simulink model "RB_KAIROS_impControl_repulsive"  (R2020b)
settings: Solver=ode4  StartTime=0.0  StopTime=t_end  FixedStep=Ts  RelTol=1e-3
values from neighbouring files (symbols this model uses):
  am = 0.3    [RB_KAIROS_ImpControl_OpSpace_quat_2020b_safety_main.m]
  am_r = 0.3    [RB_KAIROS_ImpControl_OpSpace_quat_2020b_safety_main.m]
  Kc = diag(50*ones(6,1))    [RB_KAIROS_ImpControl_OpSpace_quat_2020b_safety_main.m]
  Kp = 2*[400;400;400;400;0;0;0]    [RB_KAIROS_ImpControl_OpSpace_quat_2020b_safety_main.m]
  Kv = [1000;1000;1000;[300;300;300;300;300;300;300]]    [RB_KAIROS_ImpControl_OpSpace_quat_2020b_safety_main.m]
  model_sample_time = 0.001    [RB_KAIROS_ImpControl_OpSpace_quat_2020b_safety_main.m]
  q_dot_0 = zeros(10,1)    [RB_KAIROS_ImpControl_OpSpace_quat_2020b_safety_main.m]
  T_i = K    [RB_KAIROS_ImpControl_OpSpace_quat_2020b_safety_main.m]
  tau_ext = [0 0 0 0 0 0 0 0 0 0 0]    [RB_KAIROS_ImpControl_OpSpace_quat_2020b_safety_main.m]
  v_SMU = 10    [RB_KAIROS_ImpControl_OpSpace_quat_2020b_safety_main.m]
  vm = 0.5    [RB_KAIROS_ImpControl_OpSpace_quat_2020b_safety_main.m]
  vm_r = 0.5    [RB_KAIROS_ImpControl_OpSpace_quat_2020b_safety_main.m]
undefined symbols (not defined in the file or in its folder): DiscIntNeverNeededParam, magnitude, q_0, T_f
libraries: simulink x4, utils x4, transformations_lib x3
(part 2 of 17)

== system RB_KAIROS_impControl_repulsive/CONTROLLER /Kinematics and Dynamics/Kinematics - error representation ==
  qv : Inport
  qa : Inport  Port=2
  R_D_W_aug : Inport  Port=3
  x_dot_des : Inport  Port=4
  x_ddot_des : Inport  Port=5
  x_err : Inport  Port=6
  x_dot_err : Inport  Port=7
  qv_dot : Inport  Port=8
  qa_dot : Inport  Port=9
  Compute J_x_dot : Subsystem
  MATLAB Function1 : MATLAB Function  TreatAsAtomicUnit=on
  MATLAB Function2 : MATLAB Function  TreatAsAtomicUnit=on
  MATLAB Function3 : MATLAB Function  TreatAsAtomicUnit=on
  Terminator : Terminator
  Whole-Body Jacobian : MATLAB Function  TreatAsAtomicUnit=on
  J_x : Outport
  J_x_dot : Outport  Port=2
  vt : Outport  Port=3
  vt_dot : Outport  Port=4
  J_b : Outport  Port=5
  wires:
  qa/1 -> Compute J_x_dot/5(qa), Whole-Body Jacobian/2(qa)
  qv/1 -> Compute J_x_dot/4(qv), Whole-Body Jacobian/1(qv)
  Whole-Body Jacobian/1(J) -> MATLAB Function3/2(J_b), MATLAB Function1/1(J), J_b/1, Compute J_x_dot/1(J_b)
  MATLAB Function3/1(J_x) -> J_x/1
  Compute J_x_dot/1(J_x_dot) -> J_x_dot/1
  R_D_W_aug/1 -> MATLAB Function3/1(R_W_D_aug), Compute J_x_dot/2(R_D_W_aug), MATLAB Function2/1(R_D_W_aug)
  x_dot_des/1 -> Compute J_x_dot/3(x_dot_d), MATLAB Function2/2(x_dot_d)
  MATLAB Function2/2(vt_dot) -> vt_dot/1
  MATLAB Function2/1(vt) -> vt/1
  x_ddot_des/1 -> MATLAB Function2/3(x_ddot_d)
  x_dot_err/1 -> MATLAB Function2/5(x_dot_err)
  x_err/1 -> MATLAB Function2/4(x_err)
  MATLAB Function1/1(t) -> Terminator/1
  qv_dot/1 -> Compute J_x_dot/6(qv_dot)
  qa_dot/1 -> Compute J_x_dot/7(qa_dot)

== system RB_KAIROS_impControl_repulsive/Trajectory Generator/Subsystem1/Angle Axis Via Quaternions ==
  R : Inport
  Display : Display
  Quaternion To Angle Axis : Subsystem
  Reshape : Reshape  OutputDimensionality=Column vector (2-D)
  Selector : Selector  InputPortWidth=4  IndexOptions=Index vector (dialog)  Indices=2:4  OutputSizes=1
  Selector1 : Selector  InputPortWidth=4  IndexOptions=Index vector (dialog)  Indices=1  OutputSizes=1
  r2q : MATLAB Function  TreatAsAtomicUnit=on
  angle : Outport  VectorParamsAs1DForOutWhenUnconnected=off
  axis : Outport  Port=2  VectorParamsAs1DForOutWhenUnconnected=off
  wires:
  Quaternion To Angle Axis/2(axis) -> axis/1
  R/1 -> r2q/1(R)
  Quaternion To Angle Axis/1(angle) -> angle/1
  Selector/1 -> Reshape/1
  Selector1/1 -> Quaternion To Angle Axis/1(eta)
  r2q/1(q) -> Selector1/1, Selector/1
  Reshape/1 -> Display/1, Quaternion To Angle Axis/2(epsilon)

== system RB_KAIROS_impControl_repulsive/Trajectory Generator/Subsystem1/Normalize ==
  x : Inport
  Divide : Product  Inputs=*/
  Switch : Switch  Criteria=u2 > Threshold
  length : Subsystem
  one : Constant
  x/||x|| : Outport  VectorParamsAs1DForOutWhenUnconnected=off
  wires:
  x/1 -> Divide/1, length/1(v)
  Divide/1 -> x/||x||/1
  one/1 -> Switch/3
  length/1(|v|) -> Switch/2, Switch/1
  Switch/1 -> Divide/2

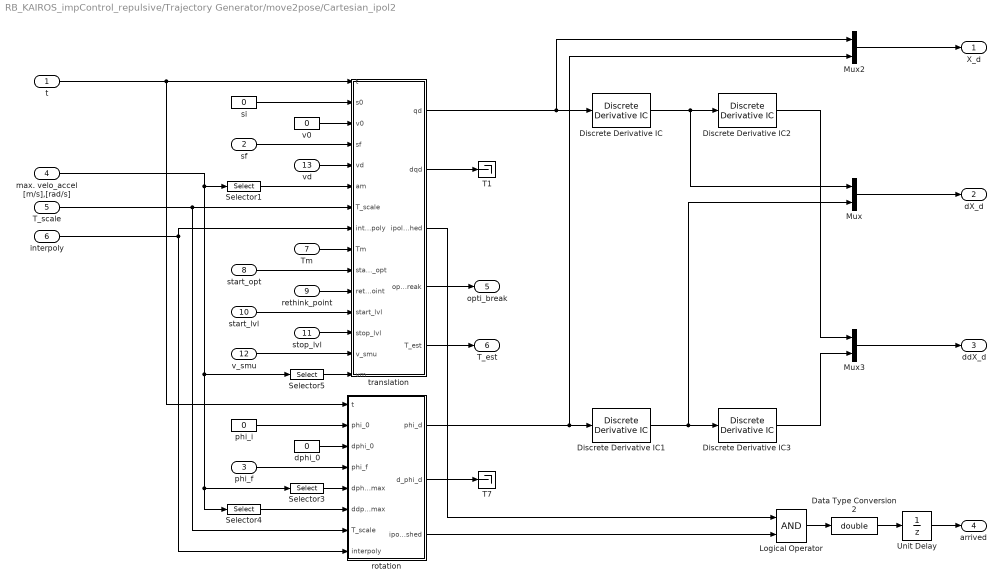
== system RB_KAIROS_impControl_repulsive/Trajectory Generator/move2pose/Cartesian_ipol2 ==
  t : Inport
  sf : Inport  Port=2
  phi_f : Inport  Port=3
  max. velo_accel [m/s],[rad/s] : Inport  Port=4
  T_scale : Inport  Port=5
  interpoly : Inport  Port=6
  Tm : Inport  Port=7
  start_opt : Inport  Port=8
  rethink_point : Inport  Port=9
  start_lvl : Inport  Port=10
  stop_lvl : Inport  Port=11
  v_smu : Inport  Port=12
  vd : Inport  Port=13
  Data Type Conversion2 : DataTypeConversion  OutDataTypeStr=double
  Discrete Derivative IC{,1..3} (4 alike) : utils/Discrete Derivative IC  model_sample_time=model_sample_time
  Logical Operator : Logic  AllPortsSameDT=off  OutDataTypeStr=boolean
  Mux : Mux  Inputs=2
  Mux2 : Mux  Inputs=2
  Mux3 : Mux  Inputs=2
  Selector1 : Selector  InputPortWidth=4  IndexOptions=Index vector (dialog)  Indices=2  OutputSizes=1
  Selector3 : Selector  InputPortWidth=4  IndexOptions=Index vector (dialog)  Indices=3  OutputSizes=1
  Selector4 : Selector  InputPortWidth=4  IndexOptions=Index vector (dialog)  Indices=4  OutputSizes=1
  Selector5 : Selector  InputPortWidth=4  IndexOptions=Index vector (dialog)  Indices=1  OutputSizes=1
  T1 : Terminator
  T7 : Terminator
  Unit Delay : UnitDelay  SampleTime=-1  HasFrameUpgradeWarning=on
  dphi_0 : Constant  Value=0
  phi_i : Constant  Value=0
  rotation : Subsystem
  si : Constant  Value=0
  translation : Subsystem
  v0 : Constant  Value=0
  X_d : Outport  VectorParamsAs1DForOutWhenUnconnected=off
  dX_d : Outport  Port=2  VectorParamsAs1DForOutWhenUnconnected=off
  ddX_d : Outport  Port=3  VectorParamsAs1DForOutWhenUnconnected=off
  arrived : Outport  Port=4  VectorParamsAs1DForOutWhenUnconnected=off
  opti_break : Outport  Port=5  VectorParamsAs1DForOutWhenUnconnected=off
  T_est : Outport  Port=6  VectorParamsAs1DForOutWhenUnconnected=off
  wires:
  sf/1 -> translation/4(sf)
  Selector1/1 -> translation/6(am)
  max. velo_accel [m/s],[rad/s]/1 -> Selector4/1, Selector3/1, Selector5/1, Selector1/1
  Data Type Conversion2/1 -> Unit Delay/1
  dphi_0/1 -> rotation/3(dphi_0)
  Selector3/1 -> rotation/5(dphi_max)
  Selector4/1 -> rotation/6(ddphi_max)
  v0/1 -> translation/3(v0)
  Mux/1 -> dX_d/1
  t/1 -> rotation/1(t), translation/1(t)
  rotation/1(phi_d) -> Discrete Derivative IC1/1, Mux2/2
  T_scale/1 -> rotation/7(T_scale), translation/7(T_scale)
  interpoly/1 -> rotation/8(interpoly), translation/8(interpoly)
  Discrete Derivative IC/1 -> Mux/1, Discrete Derivative IC2/1
  Unit Delay/1 -> arrived/1
  translation/3(ipol_finished) -> Logical Operator/1
  Logical Operator/1 -> Data Type Conversion2/1
  Mux2/1 -> X_d/1
  translation/1(qd) -> Discrete Derivative IC/1, Mux2/1
  Mux3/1 -> ddX_d/1
  Discrete Derivative IC2/1 -> Mux3/1
  Discrete Derivative IC3/1 -> Mux3/2
  Discrete Derivative IC1/1 -> Discrete Derivative IC3/1, Mux/2
  rotation/3(ipol_finished) -> Logical Operator/2
  Tm/1 -> translation/9(Tm)
  translation/4(opti_break) -> opti_break/1
  translation/5(T_est) -> T_est/1
  start_opt/1 -> translation/10(start_opt)
  rethink_point/1 -> translation/11(rethink_point)
  start_lvl/1 -> translation/12(start_lvl)
  stop_lvl/1 -> translation/13(stop_lvl)
  v_smu/1 -> translation/14(v_smu)
  phi_i/1 -> rotation/2(phi_0)
  phi_f/1 -> rotation/4(phi_f)
  rotation/2(d_phi_d) -> T7/1
  translation/2(dqd) -> T1/1
  Selector5/1 -> translation/15(vm)
  vd/1 -> translation/5(vd)
  si/1 -> translation/2(s0)

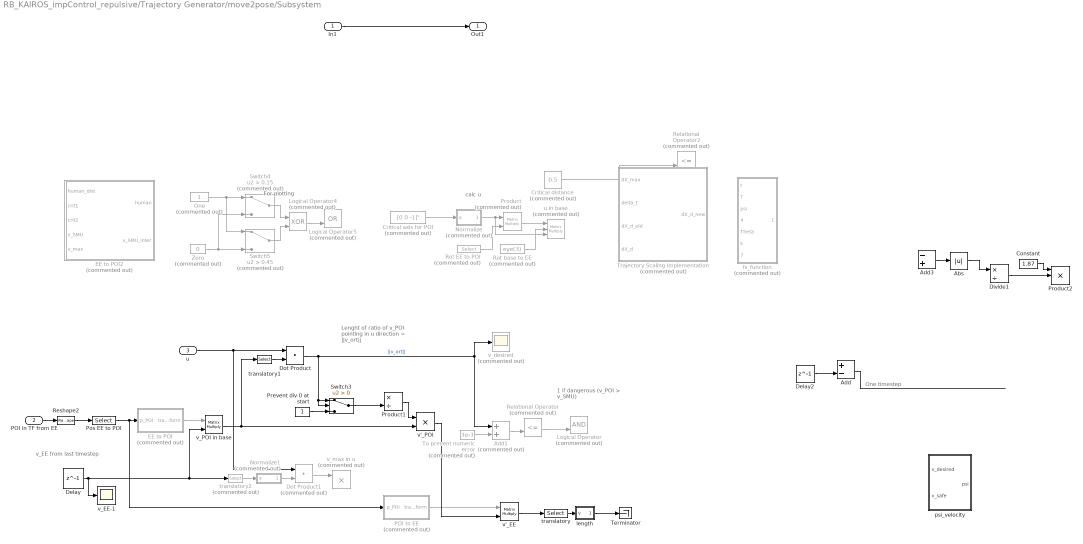
== system RB_KAIROS_impControl_repulsive/Trajectory Generator/move2pose/Subsystem ==
  note: calc u
  note: For plotting
  note: v_EE from last timestep
  note: 1 if dangerous
      | (v_POI > v_SMU)
  note: Lenght of ratio of v_POI
      | pointing in u direction
      | = ||v_ort||
  note: One timestep
  In1 : Inport
  POI in TF from EE : Inport  Port=2
  u : Inport  Port=3
  Abs : Abs
  Add : Sum  Inputs=+-
  Add1 : Sum  Commented=on
  Add3 : Sum  Inputs=-+
  Constant : Constant  Value=1.87
  Critical axis for POI : Constant  Commented=on  Value=[0 0 -1]'
  Critical distance : Constant  Commented=on  Value=0.5
  Delay : Delay  DelayLength=1
  Delay2 : Delay  DelayLength=1
  Divide1 : Product  Inputs=*/
  Dot Product : DotProduct  InputSameDT=on  OutDataTypeStr=Inherit: Inherit via internal rule
  Dot Product1 : DotProduct  Commented=on  InputSameDT=on  OutDataTypeStr=Inherit: Inherit via internal rule
  EE to POI : MATLAB Function  Commented=on  TreatAsAtomicUnit=on
  EE to POI2 : MATLAB Function  Commented=on  TreatAsAtomicUnit=on
  Logical Operator : Logic  Commented=on  AllPortsSameDT=off  OutDataTypeStr=boolean
  Logical Operator4 : Logic  Commented=on  Operator=XOR  AllPortsSameDT=off  OutDataTypeStr=boolean
  Logical Operator5 : Logic  Commented=on  Operator=OR  AllPortsSameDT=off  OutDataTypeStr=boolean
  Normalize : Subsystem  Commented=on
  Normalize1 : Subsystem  Commented=on
  One : Constant  Commented=on
  POI to EE : MATLAB Function  Commented=on  TreatAsAtomicUnit=on
  Pos EE to POI : Selector  NumberOfDimensions=2  InputPortWidth=7  IndexOptions=Index vector (dialog),Index vector (dialog)  Indices=[1:3],[4]  OutputSizes=1
  Prevent div 0 at start : Constant
  Product : Product  Commented=on  Multiplication=Matrix(*)
  Product1 : Product  Inputs=*/
  Product2 : Product  Inputs=3
  Relational Operator : RelationalOperator  Commented=on  Operator=<=  OutDataTypeStr=boolean  RndMeth=Simplest
  Relational Operator2 : RelationalOperator  Commented=on  Operator=<=  OutDataTypeStr=boolean  RndMeth=Simplest
  Reshape2 : Reshape  OutputDimensionality=Customize  OutputDimensions=[4,4]
  Rot EE to POI : Selector  Commented=on  NumberOfDimensions=2  InputPortWidth=7  IndexOptions=Index vector (dialog),Index vector (dialog)  Indices=[1:3],[1:3]  OutputSizes=1
  Rot base to EE : Constant  Commented=on  Value=eye(3)
  Switch3 : Switch  Criteria=u2 > Threshold
  Switch4 : Switch  Commented=on  Criteria=u2 > Threshold  Threshold=0.15
  Switch5 : Switch  Commented=on  Criteria=u2 > Threshold  Threshold=0.45
  Terminator : Terminator
  To prevent numeric error : Constant  Commented=on  Value=3e-3
  Trajectory Scaling Implementation : MATLAB Function  Commented=on  TreatAsAtomicUnit=on
  Zero : Constant  Commented=on  Value=0
  fs_function : MATLAB Function  Commented=on  TreatAsAtomicUnit=on
  length : Subsystem
  psi_velocity : MATLAB Function  TreatAsAtomicUnit=on
  translatory : Selector  InputPortWidth=6  IndexOptions=Index vector (dialog)  Indices=[1:3]  OutputSizes=1
  translatory1 : Selector  InputPortWidth=6  IndexOptions=Index vector (dialog)  Indices=[1:3]  OutputSizes=1
  translatory2 : Selector  Commented=on  InputPortWidth=6  IndexOptions=Index vector (dialog)  Indices=[1:3]  OutputSizes=1
  u in base : Product  Commented=on  Inputs=3  Multiplication=Matrix(*)
  v'_EE : Product  Multiplication=Matrix(*)
  v'_POI : Product
  v_EE-1 : Scope
  v_POI in base : Product  Multiplication=Matrix(*)
  v_desired : Scope  Commented=on
  v_max in u : Product  Commented=on
  Out1 : Outport  VectorParamsAs1DForOutWhenUnconnected=off
  wires:
  In1/1 -> Out1/1
  Critical axis for POI/1 -> Normalize/1(x)
  Rot EE to POI/1 -> Product/2
  Logical Operator4/1 -> Logical Operator5/2
  Product/1 -> u in base/1
  One/1 -> Switch4/1, Switch5/1
  Zero/1 -> Switch5/3, Switch4/3
  Switch4/1 -> Logical Operator4/1
  Switch5/1 -> Logical Operator4/2
  Normalize/1(x/||x||) -> u in base/3, Product/1
  Rot base to EE/1 -> u in base/2
  Critical distance/1 -> Relational Operator2/2
  Prevent div 0 at start/1 -> Switch3/3
  translatory2/1 -> Normalize1/1(x)
  Normalize1/1(x/||x||) -> Dot Product1/2
  ? -> Logical Operator/1
  ? -> v_max in u/2
  POI to EE/1(transform) -> v'_EE/1
  Add1/1 -> Relational Operator/2
  ? -> Product1/1
  v'_EE/1 -> translatory/1
  v'_POI/1 -> v'_EE/2
  EE to POI/1(transform) -> v_POI in base/1
  translatory/1 -> length/1(v)
  ? -> Relational Operator/1
  ? -> Delay/1
  v_POI in base/1 -> v'_POI/2, translatory1/1
  Dot Product1/1 -> v_max in u/1
  Delay/1 -> v_EE-1/1, v_POI in base/2, translatory2/1
  Dot Product/1 -> v_desired/1, Add1/1, Switch3/2, Switch3/1  "||v_ort||"
  translatory1/1 -> Dot Product/2
  Switch3/1 -> Product1/2
  Pos EE to POI/1 -> POI to EE/1(p_POI), EE to POI/1(p_POI)
  Reshape2/1 -> Pos EE to POI/1
  u/1 -> Dot Product/1, Dot Product1/1
  POI in TF from EE/1 -> Reshape2/1
  To prevent numeric error/1 -> Add1/2
  Product1/1 -> v'_POI/1
  length/1(|v|) -> Terminator/1
  Relational Operator/1 -> Logical Operator/2
  Delay2/1 -> Add/2
  ? -> Add/1
  ? -> Delay2/1
  Add/1 -> ?
  Abs/1 -> Divide1/1
  Constant/1 -> Product2/1
  Divide1/1 -> Product2/2
  Add3/1 -> Abs/1

== system RB_KAIROS_impControl_repulsive/CONTROLLER /Kinematics and Dynamics/Kinematics - error representation/Compute J_x_dot ==
  note: J_x_dot = R_D_W_aug*J_b_dot - R_D_W_aug*S(omega_d)_aug*J_b = R_D_W_aug*(J_b_dot - S(omega_d)_aug*J_b)
  J_b : Inport
  R_D_W_aug : Inport  Port=2
  x_dot_d : Inport  Port=3
  qv : Inport  Port=4
  qa : Inport  Port=5
  qv_dot : Inport  Port=6
  qa_dot : Inport  Port=7
  Add : Sum  Inputs=+-
  Augment matrix : MATLAB Function  TreatAsAtomicUnit=on
  MATLAB Function : MATLAB Function  TreatAsAtomicUnit=on
  MatrixMultiply : Product  Multiplication=Matrix(*)
  MatrixMultiply1 : Product  Multiplication=Matrix(*)
  S(omega) : MATLAB Function  TreatAsAtomicUnit=on
  Selector : Selector  InputPortWidth=6  IndexOptions=Index vector (dialog)  Indices=[4:6]  OutputSizes=1
  J_x_dot : Outport
  wires:
  Add/1 -> MatrixMultiply/2
  MATLAB Function/1(J_dot) -> Add/1
  MatrixMultiply1/1 -> Add/2
  x_dot_d/1 -> Selector/1
  Augment matrix/1(M_aug) -> MatrixMultiply1/1
  R_D_W_aug/1 -> MatrixMultiply/1
  qa_dot/1 -> MATLAB Function/4(qa_dot)
  Selector/1 -> S(omega)/1(v)
  S(omega)/1(S) -> Augment matrix/1(M)
  J_b/1 -> MatrixMultiply1/2
  qa/1 -> MATLAB Function/2(qa)
  qv_dot/1 -> MATLAB Function/3(qv_dot)
  MatrixMultiply/1 -> J_x_dot/1
  qv/1 -> MATLAB Function/1(qv)

== system RB_KAIROS_impControl_repulsive/Trajectory Generator/Subsystem1/Angle Axis Via Quaternions/Quaternion To Angle Axis ==
  eta : Inport
  epsilon : Inport  Port=2
  Divide : Product  Inputs=*/
  Gain : Gain  Gain=2
  Product : Product  RndMeth=Zero
  Saturation : Saturate  UpperLimit=1  LowerLimit=-1
  Sqrt : Sqrt  SaturateOnIntegerOverflow=on
  Subtract : Sum  Inputs=+-
  Switch1 : Switch  Criteria=u2 ~= 0
  Trigonometric Function : Trigonometry  Operator=acos
  dummy axis : Constant  Value=[1,0,0]
  one : Constant
  angle : Outport  VectorParamsAs1DForOutWhenUnconnected=off
  axis : Outport  Port=2  VectorParamsAs1DForOutWhenUnconnected=off
  wires:
  Divide/1 -> Switch1/1
  Switch1/1 -> axis/1
  dummy axis/1 -> Switch1/3
  Gain/1 -> Switch1/2, angle/1
  epsilon/1 -> Divide/1
  Trigonometric Function/1 -> Gain/1
  eta/1 -> Saturation/1
  Subtract/1 -> Sqrt/1
  one/1 -> Subtract/1
  Product/1 -> Subtract/2
  Sqrt/1 -> Divide/2
  Saturation/1 -> Trigonometric Function/1, Product/1, Product/2

== system RB_KAIROS_impControl_repulsive/Trajectory Generator/Subsystem1/Normalize/length ==
  v : Inport
  Abs1 : Abs
  Add : Sum  Inputs=+
  Math Function : Math  Operator=magnitude^2  SignedPower=on  SaturateOnIntegerOverflow=on
  Sqrt : Sqrt  Operator=signedSqrt  SaturateOnIntegerOverflow=on
  |v| : Outport  VectorParamsAs1DForOutWhenUnconnected=off
  wires:
  Math Function/1 -> Add/1
  Add/1 -> Sqrt/1
  v/1 -> Math Function/1
  Abs1/1 -> |v|/1
  Sqrt/1 -> Abs1/1

== system RB_KAIROS_impControl_repulsive/Trajectory Generator/move2pose/Cartesian_ipol2/rotation ==
  t : Inport
  phi_0 : Inport  Port=2
  dphi_0 : Inport  Port=3
  phi_f : Inport  Port=4
  dphi_max : Inport  Port=5
  ddphi_max : Inport  Port=6
  T_scale : Inport  Port=7
  interpoly : Inport  Port=8
  Abs1 : Abs
  Compare To Constant : simulink/Logic and Bit Operations/Compare To Constant  relop=<=  const=1e-9  OutDataTypeStr=boolean
  Data Type Conversion : DataTypeConversion  OutDataTypeStr=boolean
  Embedded MATLAB Function1 : MATLAB Function  TreatAsAtomicUnit=on
  Logical Operator2 : Logic  Operator=OR  AllPortsSameDT=off  OutDataTypeStr=boolean
  Subtract1 : Sum  Inputs=-+
  T7 : Terminator
  phi_d : Outport  VectorParamsAs1DForOutWhenUnconnected=off
  d_phi_d : Outport  Port=2  VectorParamsAs1DForOutWhenUnconnected=off
  ipol_finished : Outport  Port=3  VectorParamsAs1DForOutWhenUnconnected=off
  wires:
  ddphi_max/1 -> Embedded MATLAB Function1/6(am)
  dphi_max/1 -> Embedded MATLAB Function1/5(vm)
  dphi_0/1 -> Embedded MATLAB Function1/3(v0)
  phi_0/1 -> Embedded MATLAB Function1/2(s0)
  t/1 -> Embedded MATLAB Function1/1(t)
  Embedded MATLAB Function1/3(ddqd) -> T7/1
  interpoly/1 -> Embedded MATLAB Function1/8(interpoly)
  T_scale/1 -> Embedded MATLAB Function1/7(T_scale)
  Compare To Constant/1 -> Logical Operator2/2
  Subtract1/1 -> Abs1/1
  Abs1/1 -> Compare To Constant/1
  Logical Operator2/1 -> ipol_finished/1
  Embedded MATLAB Function1/4(ipol_finished) -> Data Type Conversion/1
  Data Type Conversion/1 -> Logical Operator2/1
  phi_f/1 -> Subtract1/2, Embedded MATLAB Function1/4(sf)
  Embedded MATLAB Function1/2(dqd) -> d_phi_d/1
  Embedded MATLAB Function1/1(qd) -> phi_d/1, Subtract1/1

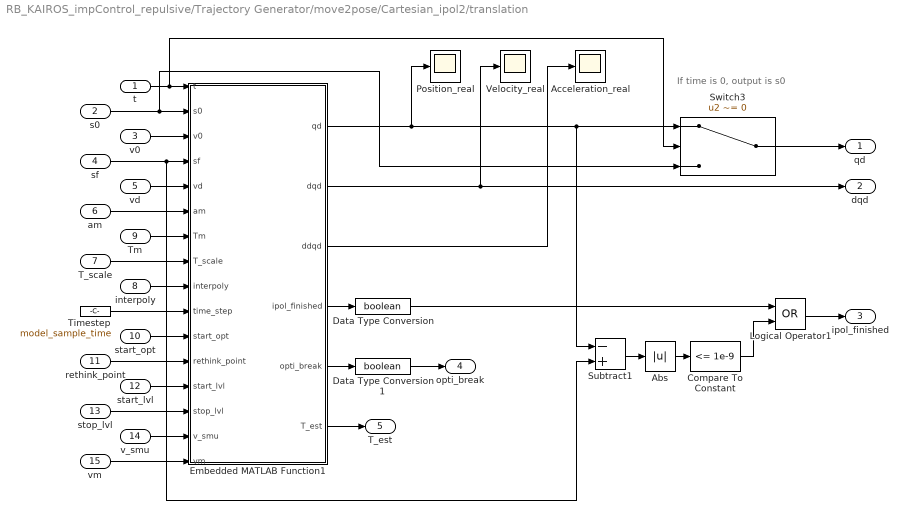
== system RB_KAIROS_impControl_repulsive/Trajectory Generator/move2pose/Cartesian_ipol2/translation ==
  note: If time is 0, output is s0
  t : Inport
  s0 : Inport  Port=2
  v0 : Inport  Port=3
  sf : Inport  Port=4
  vd : Inport  Port=5
  am : Inport  Port=6
  T_scale : Inport  Port=7
  interpoly : Inport  Port=8
  Tm : Inport  Port=9
  start_opt : Inport  Port=10
  rethink_point : Inport  Port=11
  start_lvl : Inport  Port=12
  stop_lvl : Inport  Port=13
  v_smu : Inport  Port=14
  vm : Inport  Port=15
  Abs : Abs
  Acceleration_real : Scope
  Compare To Constant : simulink/Logic and Bit Operations/Compare To Constant  relop=<=  const=1e-9  OutDataTypeStr=boolean
  Data Type Conversion : DataTypeConversion  OutDataTypeStr=boolean
  Data Type Conversion1 : DataTypeConversion  OutDataTypeStr=boolean
  Embedded MATLAB Function1 : MATLAB Function  TreatAsAtomicUnit=on
  Logical Operator1 : Logic  Operator=OR  AllPortsSameDT=off  OutDataTypeStr=boolean
  Position_real : Scope
  Subtract1 : Sum  Inputs=-+
  Switch3 : Switch  Criteria=u2 ~= 0
  Timestep : Constant  Value=model_sample_time
  Velocity_real : Scope
  qd : Outport  VectorParamsAs1DForOutWhenUnconnected=off
  dqd : Outport  Port=2  VectorParamsAs1DForOutWhenUnconnected=off
  ipol_finished : Outport  Port=3  VectorParamsAs1DForOutWhenUnconnected=off
  opti_break : Outport  Port=4  VectorParamsAs1DForOutWhenUnconnected=off
  T_est : Outport  Port=5  VectorParamsAs1DForOutWhenUnconnected=off
  wires:
  Switch3/1 -> qd/1
  Logical Operator1/1 -> ipol_finished/1
  Embedded MATLAB Function1/2(dqd) -> Velocity_real/1, dqd/1
  Embedded MATLAB Function1/1(qd) -> Switch3/1, Subtract1/1, Position_real/1
  s0/1 -> Embedded MATLAB Function1/2(s0), Switch3/3
  t/1 -> Switch3/2, Embedded MATLAB Function1/1(t)
  am/1 -> Embedded MATLAB Function1/6(am)
  vd/1 -> Embedded MATLAB Function1/5(vd)
  v0/1 -> Embedded MATLAB Function1/3(v0)
  Subtract1/1 -> Abs/1
  Compare To Constant/1 -> Logical Operator1/2
  Abs/1 -> Compare To Constant/1
  Embedded MATLAB Function1/3(ddqd) -> Acceleration_real/1
  T_scale/1 -> Embedded MATLAB Function1/8(T_scale)
  interpoly/1 -> Embedded MATLAB Function1/9(interpoly)
  Embedded MATLAB Function1/4(ipol_finished) -> Data Type Conversion/1
  Data Type Conversion/1 -> Logical Operator1/1
  Timestep/1 -> Embedded MATLAB Function1/10(time_step)
  Tm/1 -> Embedded MATLAB Function1/7(Tm)
  Embedded MATLAB Function1/5(opti_break) -> Data Type Conversion1/1
  Data Type Conversion1/1 -> opti_break/1
  Embedded MATLAB Function1/6(T_est) -> T_est/1
  start_opt/1 -> Embedded MATLAB Function1/11(start_opt)
  rethink_point/1 -> Embedded MATLAB Function1/12(rethink_point)
  start_lvl/1 -> Embedded MATLAB Function1/13(start_lvl)
  stop_lvl/1 -> Embedded MATLAB Function1/14(stop_lvl)
  v_smu/1 -> Embedded MATLAB Function1/15(v_smu)
  vm/1 -> Embedded MATLAB Function1/16(vm)
  sf/1 -> Subtract1/2, Embedded MATLAB Function1/4(sf)

== system RB_KAIROS_impControl_repulsive/Trajectory Generator/move2pose/Subsystem/Normalize ==
  x : Inport
  Divide : Product  Inputs=*/
  Switch : Switch  Criteria=u2 > Threshold
  length : Subsystem
  one : Constant
  x/||x|| : Outport  VectorParamsAs1DForOutWhenUnconnected=off
  wires:
  x/1 -> Divide/1, length/1(v)
  Divide/1 -> x/||x||/1
  one/1 -> Switch/3
  length/1(|v|) -> Switch/2, Switch/1
  Switch/1 -> Divide/2

== system RB_KAIROS_impControl_repulsive/Trajectory Generator/move2pose/Subsystem/Normalize1 ==
  x : Inport
  Divide : Product  Inputs=*/
  Switch : Switch  Criteria=u2 > Threshold
  length : Subsystem
  one : Constant
  x/||x|| : Outport  VectorParamsAs1DForOutWhenUnconnected=off
  wires:
  x/1 -> Divide/1, length/1(v)
  Divide/1 -> x/||x||/1
  one/1 -> Switch/3
  length/1(|v|) -> Switch/2, Switch/1
  Switch/1 -> Divide/2

== system RB_KAIROS_impControl_repulsive/Trajectory Generator/move2pose/Subsystem/length ==
  v : Inport
  Abs1 : Abs
  Add : Sum  Inputs=+
  Math Function : Math  Operator=magnitude^2  SignedPower=on  SaturateOnIntegerOverflow=on
  Sqrt : Sqrt  Operator=signedSqrt  SaturateOnIntegerOverflow=on
  |v| : Outport  VectorParamsAs1DForOutWhenUnconnected=off
  wires:
  Math Function/1 -> Add/1
  Add/1 -> Sqrt/1
  v/1 -> Math Function/1
  Abs1/1 -> |v|/1
  Sqrt/1 -> Abs1/1

== system RB_KAIROS_impControl_repulsive/Trajectory Generator/move2pose/Subsystem/Normalize/length ==
  v : Inport
  Add : Sum  Inputs=+
  Math Function : Math  Operator=magnitude^2  SignedPower=on  SaturateOnIntegerOverflow=on
  Math Function1 : Math  Operator=sqrt  SignedPower=on  SaturateOnIntegerOverflow=on
  |v| : Outport  VectorParamsAs1DForOutWhenUnconnected=off
  wires:
  Math Function/1 -> Add/1
  Add/1 -> Math Function1/1
  v/1 -> Math Function/1
  Math Function1/1 -> |v|/1

== system RB_KAIROS_impControl_repulsive/Trajectory Generator/move2pose/Subsystem/Normalize1/length ==
  v : Inport
  Abs1 : Abs
  Add : Sum  Inputs=+
  Math Function : Math  Operator=magnitude^2  SignedPower=on  SaturateOnIntegerOverflow=on
  Sqrt : Sqrt  Operator=signedSqrt  SaturateOnIntegerOverflow=on
  |v| : Outport  VectorParamsAs1DForOutWhenUnconnected=off
  wires:
  Math Function/1 -> Add/1
  Add/1 -> Sqrt/1
  v/1 -> Math Function/1
  Abs1/1 -> |v|/1
  Sqrt/1 -> Abs1/1

== matlab function RB_KAIROS_impControl_repulsive/Trajectory Generator/move2pose/Multicall ==
  data: human_dist input; human output; crit1 input; crit2 input; crit3 input; n_steps input; v_SMU input; v_SMU_step output; v_max input; v_human input; Tm output; v_human_opt input
function [human,v_SMU_step,Tm] = Multicall(human_dist,crit1,crit2,crit3,n_steps,v_SMU,v_max,v_human,v_human_opt)
% MULTICALL is a block which introduces several velocity levels between the
% maximum velocity and the safe velocity. Therefore it calls the adaption
% function multiple times with intermediate velocities. It has also a
% hysteresis, that means if the human leaves a region it is not directly
% the higher velocity applied. Only if the human leaves the next region the
% velocity rises again. 
% 
% The crit values determine the distances when to shift: 
% crit1 is the distance nearest to the robot, so here is v_SMU applied.
% crit2 is the distance when a human enters there, the velocity starts to
% decline
% crit3 is the largest distance since it is the hysteresis level for crit2,
% this means if the human distance is greater than crit3 the v_max is
% applied. 
% crit1 OR crit2 OR crit3 can be set to -1, then it is calculated
% automatically like:
% crit1 = crit2-crit_step*n_steps (crit_step = crit3-crit2)
% crit2 = crit3-crit_step
% crit3 = crit2+crit_step
%
% n_steps determines how many intermediate velocity levels should be
% applied, so n_steps=0 means deactivation of the intermediate levels.
% All distances are assumed to be positive values.

% Inputs:
% human_dist    current distance human-robot in meters
% crit1         nearest critical distance to robot
% crit2         level when to activate decline
% crit3         farest level to robot (deactivate all)
% n_steps       number of intermediate velocity levels
% v_SMU         low safe velocity
% v_max         high maximum velocity
% v_human       velocity of human for calc Tm, negative value means human
%               is approaching robot, positive value means human is leaving
%               If no real data is available an always positive estimate
%               can also be set here, see also next input.
% v_human_opt   Boolean; Set to 1 if v_human is real data, means with sign.
%               Set to 0 if v_human is always positive estimate, the sign
%               is estimated then from the human_distance. Actually it is
%               safe against wrong settings, except one special case: If
%               the human_dist data is noisy and the difference between two
%               measurements would indicate a negative velocity, but
%               actually the velocity is still positive. In this case the
%               code sets a negative velocity, if you don't set v_human_opt
%               to true.

% Outputs:
% human         boolean; True if human is near
% v_SMU_step    current desired velocity level
% Tm            time duration till when the adaption has to be completed

%n_steps in the code means in how many steps one adapts the velocity (so at least 1)
n_steps = n_steps+1; 

% Calculate the step sizes in distance ...
if crit1<0 % If crit1 is auto set
    crit_step = crit3-crit2;
    crit1 = crit2-crit_step*n_steps; %Assumption for crit1
elseif crit2<0 % If crit2 is auto set
    crit_step = (crit3-crit1)/(n_steps+1);
    crit2 = crit3-crit_step; %Assumption for crit2
elseif crit3<0 % If crit3 is auto set
    crit_step = (crit2-crit1)/n_steps;
    crit3 = crit2+crit_step; %Assumption for crit3
else
    crit_step = (crit2-crit1)/n_steps;
end
% ... and velocity
v_step = (v_max-v_SMU)/n_steps;

persistent human_1 v_SMU_step_1 human_trigger human_dist_1 %last_trigger 
if isempty(human_1)  %remembers the human state from last run
    if human_dist<=crit2 %only init
        human_1 = 1;
    else
        human_1 = 0;
    end
end
if isempty(v_SMU_step_1)   %remembers the v_SMU_step from last run
    if human_dist<=crit2 %only init
        v_SMU_step_1 = v_SMU;
    else
        v_SMU_step_1 = v_max; 
    end
end
if isempty(human_trigger)
    human_trigger = 0;    %remembers the human_trigger, so which border is triggered
end
if isempty(human_dist_1)
    human_dist_1 = human_dist;    %remembers the human_distance from last run, to auto calc sign(v_human)
end

% if v_human is an estimate without sign the sign is estimated from two
% human_distances, but this might cause errors, due to noise in human_dist.
% Thats why the option is still there. But if someone sends real data
% (especially negative values) and forgets to set option true, this would
% also cause problems, therefore if v_human is negative it is not again
% multiplied (what would make it positive!)
if v_human_opt == false && v_human>0
    v_human = v_human*sign(human_dist-human_dist_1);
end

% First set old values, if no changes occur
human = human_1;
v_SMU_step = v_SMU_step_1;

% compute borders
borders = zeros(n_steps+1,1);
for i=0:n_steps
   borders(i+1) = crit2-i*crit_step; %compute distance borders between crit1 and crit2 (inclusive both)
end

borders2 = borders+ones(size(borders))*crit_step; %shift to crit3
borders2(1) = crit3; %override for crit3, if crit3~=Assumption
region = xor(borders<human_dist,borders2<human_dist); %region is a vector with a single 1 at that region in which the human is currently
[region_max,ind] = max(region); %search for index of region

if region_max==0 %But if no 1 is contained in region, the human is somewhere else
    if human_dist>crit3 %human far away
        ind = 0;
    elseif human_dist<=crit1 %human very close
        ind = n_steps+1;
    end
end

% Slow down transition 
if ind>=2 && human_trigger<ind-1 %if human is at least in second region and this region is not triggered jet
    human = 1; % activate human bit
    human_trigger = ind-1;
    
% Speed up transition
elseif ind<=n_steps-1 && human_trigger>ind %if human is at least two steps away from robot and this region was triggered somewhen
    if ind==0 %if human is far away; switch adaption of
        human = 0;
        v_SMU_step = v_max;
    else
        human = 1;
    end
    human_trigger = ind;
end

%calculate new velocity, for the current triggered border
v_SMU_step = v_max - v_step*human_trigger; 

% Calc Tm
inf_time = 10000;
if human_dist<=crit1 %human very close => No time for adaption left
    Tm = 0;
elseif human_dist>crit3 %human very far => inf time for adaption left
    Tm = inf_time;
else
    if abs(v_human)<=1e-4 %human is nearly standing still => inf time to adapt
        Tm = inf_time;
    elseif v_human>0 %human is leaving => inf time to adapt
        Tm = inf_time;
    else
        if human_trigger==0
            crit_th = borders(2); %outside crit2 the nearest border for adapt is the next nearer border seen from crit2
        else
            crit_th = borders(human_trigger+1); %in general set crit threshold to next nearer border
        end
        % abs(v) because velocity is negative here
        Tm = (human_dist-crit_th)/abs(v_human); 
        
    end
end

% remeber current settings
human_1 = human;
v_SMU_step_1 = v_SMU_step;
human_dist_1 = human_dist;

end %end of function

%% Two steps version
% % Sequence of ifs is important, if greater steps occur!!
% % Slow down transitions
% if human_dist < crit2-crit_step*2 && human_trigger(3) == 0
%     v_SMU_step = v_max - v_step*3;
%     human = 1;
%     human_trigger(3) = 1;
%     human_trigger(2) = 1;
%     human_trigger(1) = 1;
% elseif human_dist < crit2-crit_step && human_trigger(2) == 0
%     v_SMU_step = v_max - v_step*2;
%     human = 1;
%     human_trigger(2) = 1;
%     human_trigger(1) = 1;
% elseif human_dist < crit2 && human_trigger(1) == 0
%     v_SMU_step = v_max - v_step;
%     human = 1;
%     human_trigger(1) = 1;
%     
% % Speed up transitions
% elseif human_dist > crit3 && human_trigger(1) == 1
%     v_SMU_step = v_max;
%     human = 0;
%     human_trigger(1) = 0; 
%     human_trigger(2) = 0;
%     human_trigger(3) = 0;
% elseif human_dist > crit2 && human_trigger(2) == 1
%     v_SMU_step = v_max - v_step;
%     human = 1;
%     human_trigger(2) = 0;
%     human_trigger(3) = 0;  
% elseif human_dist > crit2-crit_step && human_trigger(3) == 1 %ind ==2
%     v_SMU_step = v_max - v_step*2;
%     human = 1;
%     human_trigger(3) = 0;
%     
% end


%% Dynamic version; not working
% persistent region_1 human_1 v_SMU_step_1
% if isempty(region_1)
%     region_1 = zeros(n_steps+1,1);    %remembers the psi from last run
% end
% if isempty(human_1)
%     human_1 = 0;    %remembers the psi from last run
% end
% if isempty(v_SMU_step_1)
%     v_SMU_step_1 = v_max;    %remembers the psi from last run
% end
% 
% crit_step = (crit2-crit1)/n_steps;
% crit3 = crit2+crit_step;
% 
% v_step = (v_max-v_SMU)/n_steps;
% 
% region = zeros(n_steps+1,1);
% borders = zeros(n_steps+1,1);
% 
% if human_dist >= crit3 %Human far away
%     human = 0;
%     v_SMU_step = v_SMU;
% elseif human_dist <= crit1 %Human very close
%     human = 1;
%     v_SMU_step = v_SMU;
% else
%     % the complex part inbetween...
%     
%     for i=0:n_steps
%        borders(i+1) = crit2-i*crit_step; %compute distance borders between crit1 and crit2 (inclusive both)
%     end
%     
%     borders2 = borders+ones(size(borders))*crit_step; %shift to crit3
%     region = xor(borders<human_dist,borders2<human_dist); %region is a vector with a single 1 at that region in which the human is currently
%     [~,ind] = max(region);
%     [~,ind_1] = max(region_1);
% 
%     if ind == ind_1 %No change = human in same region
%         human = human_1;
%         v_SMU_step = v_SMU_step_1;
%     elseif ind > ind_1 %steps closer
%         human = 1;
%         v_SMU_step = v_max-v_step;        
%     elseif ind < ind_1 %steps away
%         
%     end
%            
%     
%     
%     region_1 = region;
% end

== matlab function RB_KAIROS_impControl_repulsive/CONTROLLER /Kinematics and Dynamics/Compute quantities ==
  data: M input; C input; Lambda output; mu output; J_x_T output; J_x input; J_x_d input; J_x_i output
function [Lambda, mu, J_x_T, J_x_i] = configuration_to_cartesian(M,C,J_x,J_x_d)

%Converts Mass Matrix, Coriolis/Centrifugal Matrix to Cartesian space
%representation

%M_i = inv(M);

%For redundant robots, it is not possible to direclty get the Mass Matrix
%in the cartesia space, thus a "pseudo Mass Matrix" is provided (this is 
%valid also for non-redundant robots):
Lambda_i = J_x/M*J_x';

%Here pinv is used for ensuring an inverse also in case of singular
%matrices. This is particularly useful when the selected Jacobian is
%considering only the arm or the vehicle.
Lambda = pinv(Lambda_i);

%Dynamically consistent pseudo-inverse:
J_x_i = M\J_x'*Lambda; 

%Cartesian Coriolis/Centrifugal Matrix
mu = J_x_i'*(C-M*J_x_i*J_x_d)*J_x_i;

%transpose of the Jacobian
J_x_T = J_x';
